simulink model "SysConfStateMachTest"  (R2012b)
settings: Solver=ode1  StartTime=0.0  StopTime=Inf  FixedStep=Tsample_simulink  RelTol=1e-3
PostLoadFcn:
  | , if any(exist('dsrtsu_mdlpostloadfcn', 'file') == [2, 3, 6]), try dsrtsu_mdlpostloadfcn('Execute', bdroot); catch fprintf('Error in PostLoadFcn (dsrtsu_mdlpostloadfcn) for model "%s":\n %s\n', bdroot, lasterr); end, end,
values from neighbouring files (symbols this model uses):
  Tsample_simulink = Ts/10    (= 2e-05)    [load_system_parameters.m]
libraries: simulink_extras x2
(part 8 of 9)

== stateflow chart SysConfStateMachTest/System Configuration State Machine ==
  state Off
    entry:
    IGBT_Top_State = 0
    IGBT_Bot_State = 0
    AutomaticController = 0
    ChargingRelay = 0
    DischargingRelay = 0
    BatteryRelay = 0
    UltracapacitorRelay = 0
  state DischargingRail
    during:
    IGBT_Top_State = 0
    IGBT_Bot_State = 0
    AutomaticController = 0
    ChargingRelay = 0
    DischargingRelay = 1
    BatteryRelay = 0
    UltracapacitorRelay = 0
  state ChargingRail
    during:
    IGBT_Top_State = 0
    IGBT_Bot_State = 0
    AutomaticController = 0
    ChargingRelay = 1
    DischargingRelay = 0
    BatteryRelay = 0
    UltracapacitorRelay = 0
  state FinishedCharging
    during:
    IGBT_Top_State = 0
    IGBT_Bot_State = 0
    AutomaticController = 0
    ChargingRelay = 0
    DischargingRelay = 0
    BatteryRelay = 0
    UltracapacitorRelay = 0
  state AutomaticControlMode
    during:
    IGBT_Top_State = 1
    IGBT_Bot_State = 1
    AutomaticController = 1
    ChargingRelay = 0
    DischargingRelay = 0
    BatteryRelay = 1
    UltracapacitorRelay = 1
  state ManualBuckMode
    during:
    IGBT_Top_State = 2
    IGBT_Bot_State = 0
    AutomaticController = 0
    ChargingRelay = 0
    DischargingRelay = 0
    BatteryRelay = 1
    UltracapacitorRelay = 1
  state ManualBoostMode
    during:
    IGBT_Top_State = 0
    IGBT_Bot_State = 2
    AutomaticController = 0
    ChargingRelay = 0
    DischargingRelay = 0
    BatteryRelay = 1
    UltracapacitorRelay = 1
  (default) -> Off
  DischargingRail -> Off [order 2] : [Vrail <= Vrail_rated*0.15 && abs(dVrail_dT) <= 0.1]
  Off -> ChargingRail : [TurnOnSystem == 1 && Error == 0]
  DischargingRail -> ChargingRail [order 1] : [TurnOnSystem == 1 && Error == 0]
  ChargingRail -> DischargingRail [order 2] : [Error == 1 || TurnOnSystem == 0]
  FinishedCharging -> DischargingRail [order 2] : [Error == 1 || TurnOnSystem == 0]
  ChargingRail -> FinishedCharging [order 1] : [Vrail >= Vrail_rated*0.85 && abs(dVrail_dT) <= 0.1]
  ManualBuckMode -> DischargingRail [order 3] : [Error == 1 || TurnOnSystem == 0]
  ManualBoostMode -> DischargingRail [order 3] : [Error == 1 || TurnOnSystem == 0]
  AutomaticControlMode -> DischargingRail [order 3] : [Error == 1 || TurnOnSystem == 0]
  FinishedCharging -> ManualBuckMode [order 4] : [EnableAutomaticControl == 0 ...
      | && ManualControlBuckMode == 1]
  FinishedCharging -> ManualBoostMode [order 3] : [EnableAutomaticControl == 0 ...
      | && ManualControlBuckMode == 0]
  FinishedCharging -> AutomaticControlMode [order 1] : [EnableAutomaticControl == 1]
  ManualBoostMode -> AutomaticControlMode [order 2] : [EnableAutomaticControl == 1]
  ManualBuckMode -> ManualBoostMode [order 1] : [ManualControlBuckMode == 0]
  AutomaticControlMode -> ManualBoostMode [order 1] : [EnableAutomaticControl == 0 &&...
      | ManualControlBuckMode == 0]
  ManualBoostMode -> ManualBuckMode [order 1] : [ManualControlBuckMode == 1]
  AutomaticControlMode -> ManualBuckMode [order 2] : [EnableAutomaticControl == 0 && ManualControlBuckMode == 1]
  ManualBuckMode -> AutomaticControlMode [order 2] : [EnableAutomaticControl == 1]
  data: TurnOnSystem input; EnableAutomaticControl input; ManualControlBuckMode input; Error input; IGBT_Top_State output; IGBT_Bot_State output; Vrail input; dVrail_dT input; Vrail_rated input; AutomaticController output boolean; UltracapacitorRelay output double; ChargingRelay output double; DischargingRelay output double; BatteryRelay output double
